simulink model "test"  (R2015b)
settings: Solver=FixedStepDiscrete  StartTime=0.0  StopTime=10.0  FixedStep=0.0005  RelTol=1e-3
undefined symbols (not defined in the file): I_AN03_5V, I_AN11_5V, I_SW11_H, O_SW12_HS1A
libraries: ec5744lib x12, simulink x1
settings Model: Creator=28061  LastModifiedBy=VICTOR7
settings OptimizationCC: DefaultParameterBehavior=Inlined  InlineInvariantSignals=on  ExpressionFolding=off  RollThreshold=9  StateBitsets=on  DataBitsets=on  ZeroExternalMemoryAtStartup=off  ZeroInternalMemoryAtStartup=off  EfficientFloat2IntCast=on  LifeSpan=1
settings DebuggingCC: InheritedTsInSrcMsg=none
settings HardwareCC: ProdBitPerPointer=32  ProdLargestAtomicInteger=Long  ProdLargestAtomicFloat=Double  ProdEndianess=BigEndian  ProdWordSize=32  ProdHWDeviceType=Freescale MPC5500
settings RTWCC: SystemTargetFile=ec5744.tlc  MakeCommand=make_rtw optimized_fixed_point=1  GenerateMakefile=off  TemplateMakefile=ec5744_lcc.tmf  PostCodeGenCommand=ec5744_pst_s2(buildInfo)  Description=Target for EC5744  GenerateReport=on  IncludeHyperlinkInReport=on  LaunchReport=on
settings CodeAppCC: IgnoreCustomStorageClasses=off
settings STFCustomTargetCC: ModelReferenceCompliant=off  ConcurrentExecutionCompliant=off  IncludeMdlTerminateFcn=off  GeneratePreprocessorConditionals=Use local settings  CombineOutputUpdateFcns=on  SuppressErrorStatus=on  ERTCustomFileBanners=on  SupportContinuousTime=off  SupportNonInlinedSFcns=off  SupportVariableSizeSignals=on  MATLABClassNameForMDSCustomization=Simulink.SoftwareTarget.ERTCustomization  CPPClassGenCompliant=off  GRTInterface=off  SystemTargetFile=ec5744.tlc
settings ERTTargetCC: ModelReferenceCompliant=off  ParMdlRefBuildCompliant=off  CompOptLevelCompliant=off  ConcurrentExecutionCompliant=off  IncludeMdlTerminateFcn=off  SuppressErrorStatus=on  ERTFirstTimeCompliant=off  SupportVariableSizeSignals=on  ModelStepFunctionPrototypeControlCompliant=off  CPPClassGenCompliant=off  UseToolchainInfoCompliant=off  GenerateASAP2=on  InlinedParameterPlacement=NonHierarchical  ERTSrcFileBannerTemplate=ec5744_code_template.cgt  ERTHdrFileBannerTemplate=ec5744_code_template.cgt  ERTDataSrcFileTemplate=ec5744_code_template.cgt  ERTDataHdrFileTemplate=ec5744_code_template.cgt  ERTCustomFileTemplate=ec5744_file_process.tlc

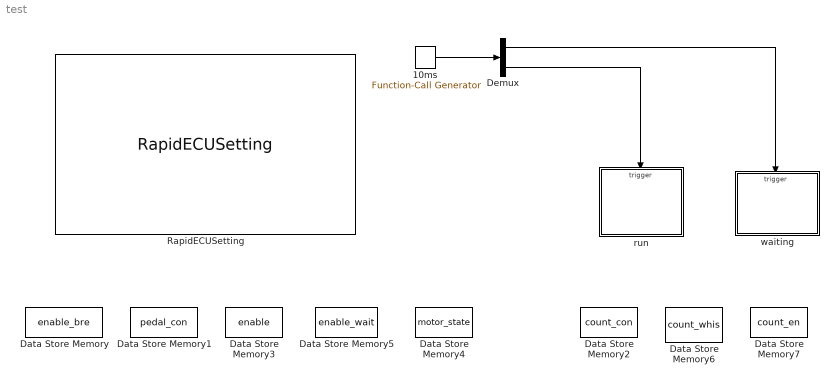
== system test ==
  10ms : simulink/Ports & Subsystems/Function-Call Generator  sample_time=0.01  numberOfIterations=1
  Data Store Memory : DataStoreMemory  DataStoreName=enable_bre  ReadBeforeWriteMsg=warning  WriteAfterWriteMsg=warning  WriteAfterReadMsg=warning
  Data Store Memory1 : DataStoreMemory  DataStoreName=pedal_con  ReadBeforeWriteMsg=warning  WriteAfterWriteMsg=warning  WriteAfterReadMsg=warning
  Data Store Memory2 : DataStoreMemory  DataStoreName=count_con  ReadBeforeWriteMsg=warning  WriteAfterWriteMsg=warning  WriteAfterReadMsg=warning  OutDataTypeStr=double
  Data Store Memory3 : DataStoreMemory  DataStoreName=enable  ReadBeforeWriteMsg=warning  WriteAfterWriteMsg=warning  WriteAfterReadMsg=warning  OutDataTypeStr=boolean
  Data Store Memory4 : DataStoreMemory  DataStoreName=motor_state  ReadBeforeWriteMsg=warning  WriteAfterWriteMsg=warning  WriteAfterReadMsg=warning
  Data Store Memory5 : DataStoreMemory  DataStoreName=enable_wait  ReadBeforeWriteMsg=warning  WriteAfterWriteMsg=warning  WriteAfterReadMsg=warning  OutDataTypeStr=boolean
  Data Store Memory6 : DataStoreMemory  DataStoreName=count_whis  ReadBeforeWriteMsg=warning  WriteAfterWriteMsg=warning  WriteAfterReadMsg=warning  OutDataTypeStr=double
  Data Store Memory7 : DataStoreMemory  DataStoreName=count_en  ReadBeforeWriteMsg=warning  WriteAfterWriteMsg=warning  WriteAfterReadMsg=warning  OutDataTypeStr=double
  Demux : Demux  Outputs=2
  RapidECUSetting : ec5744lib/RapidECU_U3/RapidECUSetting
  run : Subsystem
  waiting : Subsystem
  wires:
  10ms/1 -> Demux/1
  Demux/2 -> run/Trigger
  Demux/1 -> waiting/Trigger

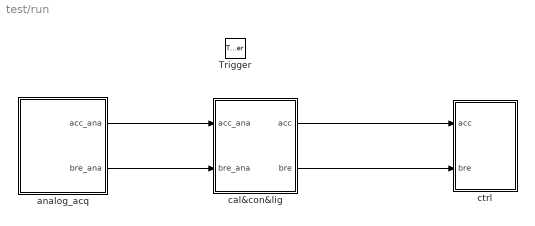
== system test/run ==
  Trigger : TriggerPort  TriggerType=function-call  PortDimensions=1
  analog_acq : Subsystem
  cal&con&lig : Subsystem
  ctrl : Subsystem
  wires:
  analog_acq/2(bre_ana) -> cal&con&lig/2(bre_ana)
  analog_acq/1(acc_ana) -> cal&con&lig/1(acc_ana)
  cal&con&lig/1(acc) -> ctrl/1(acc)
  cal&con&lig/2(bre) -> ctrl/2(bre)

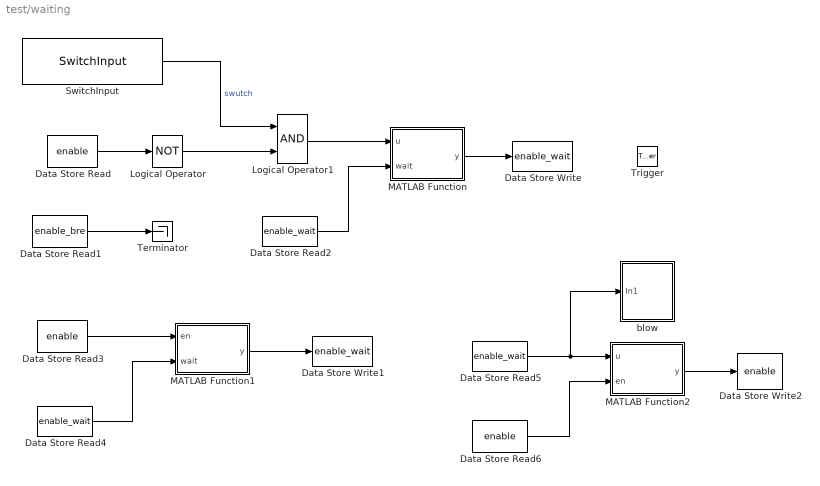
== system test/waiting ==
  Trigger : TriggerPort  TriggerType=function-call  PortDimensions=1
  Data Store Read : DataStoreRead  DataStoreName=enable
  Data Store Read1 : DataStoreRead  DataStoreName=enable_bre
  Data Store Read2 : DataStoreRead  DataStoreName=enable_wait
  Data Store Read3 : DataStoreRead  DataStoreName=enable
  Data Store Read4 : DataStoreRead  DataStoreName=enable_wait
  Data Store Read5 : DataStoreRead  DataStoreName=enable_wait
  Data Store Read6 : DataStoreRead  DataStoreName=enable
  Data Store Write : DataStoreWrite  DataStoreName=enable_wait
  Data Store Write1 : DataStoreWrite  DataStoreName=enable_wait
  Data Store Write2 : DataStoreWrite  DataStoreName=enable
  Logical Operator : Logic  Operator=NOT  AllPortsSameDT=off  OutDataTypeStr=boolean
  Logical Operator1 : Logic  AllPortsSameDT=off  OutDataTypeStr=boolean
  MATLAB Function : MATLAB Function  TreatAsAtomicUnit=on
  MATLAB Function1 : MATLAB Function  TreatAsAtomicUnit=on
  MATLAB Function2 : MATLAB Function  TreatAsAtomicUnit=on
  SwitchInput : ec5744lib/RapidECU_U3/01BasicInput/SwitchInput  channel=44:I_SW11_H  sampletime=-1
  Terminator : Terminator
  blow : Subsystem
  wires:
  Logical Operator/1 -> Logical Operator1/2
  MATLAB Function/1(y) -> Data Store Write/1
  Data Store Read6/1 -> MATLAB Function2/2(en)
  Logical Operator1/1 -> MATLAB Function/1(u)
  Data Store Read2/1 -> MATLAB Function/2(wait)
  Data Store Read3/1 -> MATLAB Function1/1(en)
  Data Store Read5/1 -> blow/1(In1), MATLAB Function2/1(u)
  SwitchInput/1 -> Logical Operator1/1  "swutch"
  Data Store Read4/1 -> MATLAB Function1/2(wait)
  Data Store Read/1 -> Logical Operator/1
  MATLAB Function1/1(y) -> Data Store Write1/1
  MATLAB Function2/1(y) -> Data Store Write2/1
  Data Store Read1/1 -> Terminator/1

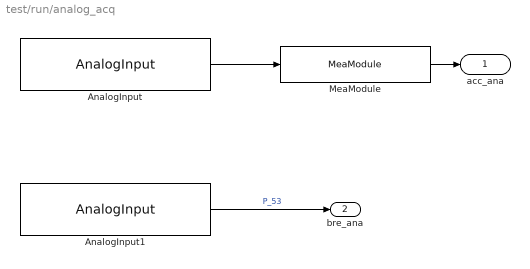
== system test/run/analog_acq ==
  AnalogInput : ec5744lib/RapidECU_U3B/01BasicInput/AnalogInput  channel=52:I_AN03_5V  sampletime=-1
  AnalogInput1 : ec5744lib/RapidECU_U3/01BasicInput/AnalogInput  channel=71:I_AN11_5V  sampletime=-1
  MeaModule : ec5744lib/RapidECU_U3B/07Calibration/MeaModule  signal=ECMeaVar1
  acc_ana : Outport
  bre_ana : Outport  Port=2
  wires:
  AnalogInput1/1 -> bre_ana/1  "P_53"
  MeaModule/1 -> acc_ana/1
  AnalogInput/1 -> MeaModule/1

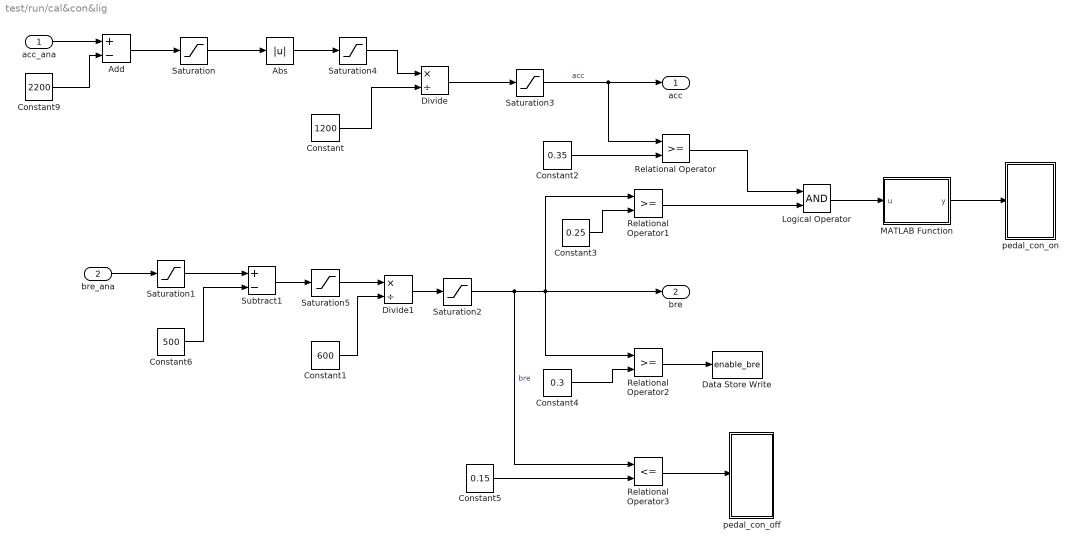
== system test/run/cal&con&lig ==
  acc_ana : Inport
  bre_ana : Inport  Port=2
  Abs : Abs
  Add : Sum  Inputs=+-
  Constant : Constant  Value=1200
  Constant1 : Constant  Value=600
  Constant2 : Constant  Value=0.35
  Constant3 : Constant  Value=0.25
  Constant4 : Constant  Value=0.3
  Constant5 : Constant  Value=0.15
  Constant6 : Constant  Value=500
  Constant9 : Constant  Value=2200
  Data Store Write : DataStoreWrite  DataStoreName=enable_bre
  Divide : Product  Inputs=*/
  Divide1 : Product  Inputs=*/
  Logical Operator : Logic  AllPortsSameDT=off  OutDataTypeStr=boolean
  MATLAB Function : MATLAB Function  TreatAsAtomicUnit=on
  Relational Operator : RelationalOperator  OutDataTypeStr=boolean
  Relational Operator1 : RelationalOperator  OutDataTypeStr=boolean
  Relational Operator2 : RelationalOperator  OutDataTypeStr=boolean
  Relational Operator3 : RelationalOperator  Operator=<=  OutDataTypeStr=boolean
  Saturation : Saturate  UpperLimit=0  LowerLimit=-1200
  Saturation1 : Saturate  UpperLimit=2466  LowerLimit=1533
  Saturation2 : Saturate  UpperLimit=1  LowerLimit=0
  Saturation3 : Saturate  UpperLimit=1  LowerLimit=0
  Saturation4 : Saturate  UpperLimit=1200  LowerLimit=0
  Saturation5 : Saturate  UpperLimit=933  LowerLimit=0
  Subtract1 : Sum  Inputs=+-
  pedal_con_off : Subsystem
  pedal_con_on : Subsystem
  acc : Outport
  bre : Outport  Port=2
  wires:
  Constant3/1 -> Relational Operator1/2
  Relational Operator1/1 -> Logical Operator/2
  Relational Operator/1 -> Logical Operator/1
  Constant5/1 -> Relational Operator3/2
  Relational Operator2/1 -> Data Store Write/1
  Constant4/1 -> Relational Operator2/2
  Relational Operator3/1 -> pedal_con_off/Enable
  MATLAB Function/1(y) -> pedal_con_on/Enable
  Logical Operator/1 -> MATLAB Function/1(u)
  Constant1/1 -> Divide1/2
  Constant/1 -> Divide/2
  Divide1/1 -> Saturation2/1
  Saturation2/1 -> Relational Operator3/1, bre/1, Relational Operator2/1, Relational Operator1/1  "bre"
  Constant2/1 -> Relational Operator/2
  bre_ana/1 -> Saturation1/1
  Divide/1 -> Saturation3/1
  Saturation1/1 -> Subtract1/1
  Constant6/1 -> Subtract1/2
  Subtract1/1 -> Saturation5/1
  Saturation5/1 -> Divide1/1
  Constant9/1 -> Add/2
  acc_ana/1 -> Add/1
  Add/1 -> Saturation/1
  Saturation/1 -> Abs/1
  Abs/1 -> Saturation4/1
  Saturation4/1 -> Divide/1
  Saturation3/1 -> Relational Operator/1, acc/1  "acc"

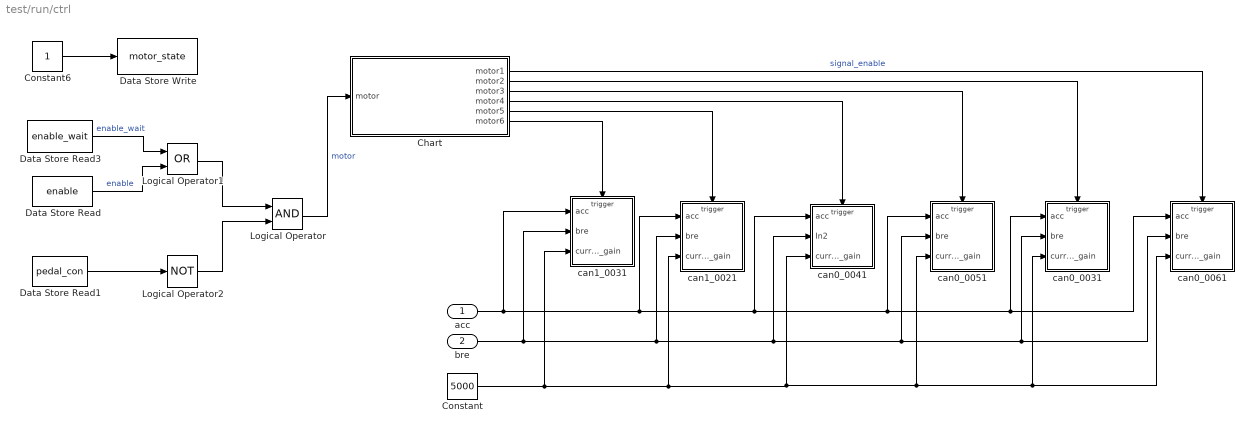
== system test/run/ctrl ==
  acc : Inport
  bre : Inport  Port=2
  Chart : Stateflow chart  TreatAsAtomicUnit=on
  Constant : Constant  Value=5000
  Constant6 : Constant
  Data Store Read : DataStoreRead  DataStoreName=enable
  Data Store Read1 : DataStoreRead  DataStoreName=pedal_con
  Data Store Read3 : DataStoreRead  DataStoreName=enable_wait
  Data Store Write : DataStoreWrite  DataStoreName=motor_state
  Logical Operator : Logic  AllPortsSameDT=off  OutDataTypeStr=boolean
  Logical Operator1 : Logic  Operator=OR  AllPortsSameDT=off  OutDataTypeStr=boolean
  Logical Operator2 : Logic  Operator=NOT  AllPortsSameDT=off  OutDataTypeStr=boolean
  can0_0031 : Subsystem
  can0_0041 : Subsystem
  can0_0051 : Subsystem
  can0_0061 : Subsystem
  can1_0021 : Subsystem
  can1_0031 : Subsystem
  wires:
  Data Store Read3/1 -> Logical Operator1/1  "enable_wait"
  Data Store Read/1 -> Logical Operator1/2  "enable"
  Logical Operator1/1 -> Logical Operator/1
  Data Store Read1/1 -> Logical Operator2/1
  Logical Operator2/1 -> Logical Operator/2
  Constant6/1 -> Data Store Write/1
  acc/1 -> can1_0031/1(acc), can0_0031/1(acc), can0_0061/1(acc), can0_0051/1(acc), can0_0041/1(acc), can1_0021/1(acc)
  bre/1 -> can1_0031/2(bre), can0_0061/2(bre), can0_0031/2(bre), can0_0051/2(bre), can0_0041/2(In2), can1_0021/2(bre)
  Chart/1(motor1) -> can0_0061/Trigger  "signal_enable"
  Chart/2(motor2) -> can0_0031/Trigger
  Chart/3(motor3) -> can0_0051/Trigger
  Chart/4(motor4) -> can0_0041/Trigger
  Logical Operator/1 -> Chart/1(motor)  "motor"
  Constant/1 -> can1_0031/3(current_gain), can0_0061/3(current_gain), can0_0031/3(current_gain), can0_0051/3(current_gain), can0_0041/3("current_gain "), can1_0021/3(current_gain)
  Chart/5(motor5) -> can1_0021/Trigger
  Chart/6(motor6) -> can1_0031/Trigger

== system test/waiting/blow ==
  In1 : Inport
  Chart : Stateflow chart  TreatAsAtomicUnit=on
  Data Type Conversion : DataTypeConversion  OutDataTypeStr=boolean
  PowerDriverSwitch(HS)2 : ec5744lib/RapidECU_U3/02PowerDriverSwitch/PowerDriverSwitch(HS)  channel=114:O_SW12_HS1A  sampletime=-1
  wires:
  In1/1 -> Data Type Conversion/1
  Data Type Conversion/1 -> Chart/1(blow_signal)
  Chart/1(blow_enable) -> PowerDriverSwitch(HS)2/1  "blow"

== system test/run/cal&con&lig/pedal_con_off ==
  Enable : EnablePort
  Constant6 : Constant  Value=0
  Data Store Write1 : DataStoreWrite  DataStoreName=pedal_con
  wires:
  Constant6/1 -> Data Store Write1/1

== system test/run/cal&con&lig/pedal_con_on ==
  Enable : EnablePort
  Constant4 : Constant
  Data Store Write : DataStoreWrite  DataStoreName=pedal_con
  wires:
  Constant4/1 -> Data Store Write/1

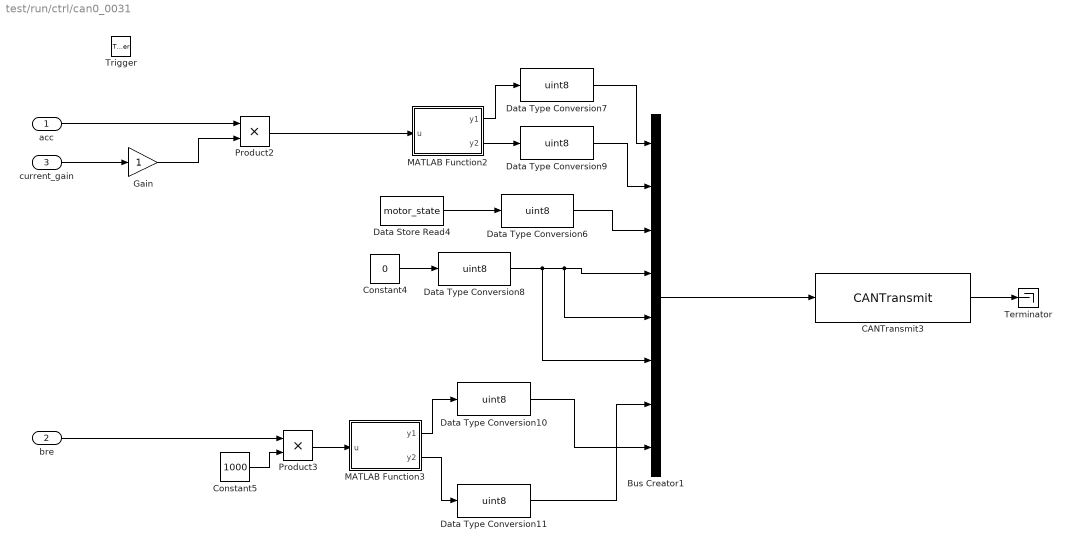
== system test/run/ctrl/can0_0031 ==
  acc : Inport
  bre : Inport  Port=2
  current_gain : Inport  Port=3
  Trigger : TriggerPort  PortDimensions=1
  Bus Creator1 : BusCreator  Inputs=8
  CANTransmit3 : ec5744lib/RapidECU_U3B/04CANCommunication/CANTransmit  canmodule=0  canbuffer=63  canmessageid=hex2dec('0031')  canmessagetype=Standard(11-bit ID)  datalength=8  sampletime=-1
  Constant4 : Constant  Value=0
  Constant5 : Constant  Value=1000
  Data Store Read4 : DataStoreRead  DataStoreName=motor_state
  Data Type Conversion{6..11} (6 alike) : DataTypeConversion  OutDataTypeStr=uint8
  Gain : Gain
  MATLAB Function2 : MATLAB Function  TreatAsAtomicUnit=on
  MATLAB Function3 : MATLAB Function  TreatAsAtomicUnit=on
  Product2 : Product
  Product3 : Product
  Terminator : Terminator
  wires:
  acc/1 -> Product2/1
  MATLAB Function3/2(y2) -> Data Type Conversion11/1
  Constant4/1 -> Data Type Conversion8/1
  Constant5/1 -> Product3/2
  Data Type Conversion8/1 -> Bus Creator1/4, Bus Creator1/5, Bus Creator1/6
  Data Type Conversion6/1 -> Bus Creator1/3
  Data Type Conversion7/1 -> Bus Creator1/1
  Data Store Read4/1 -> Data Type Conversion6/1
  Data Type Conversion9/1 -> Bus Creator1/2
  MATLAB Function2/1(y1) -> Data Type Conversion7/1
  Data Type Conversion11/1 -> Bus Creator1/7
  bre/1 -> Product3/1
  MATLAB Function2/2(y2) -> Data Type Conversion9/1
  Product3/1 -> MATLAB Function3/1(u)
  Data Type Conversion10/1 -> Bus Creator1/8
  Product2/1 -> MATLAB Function2/1(u)
  MATLAB Function3/1(y1) -> Data Type Conversion10/1
  Bus Creator1/1 -> CANTransmit3/1
  current_gain/1 -> Gain/1
  Gain/1 -> Product2/2
  CANTransmit3/1 -> Terminator/1

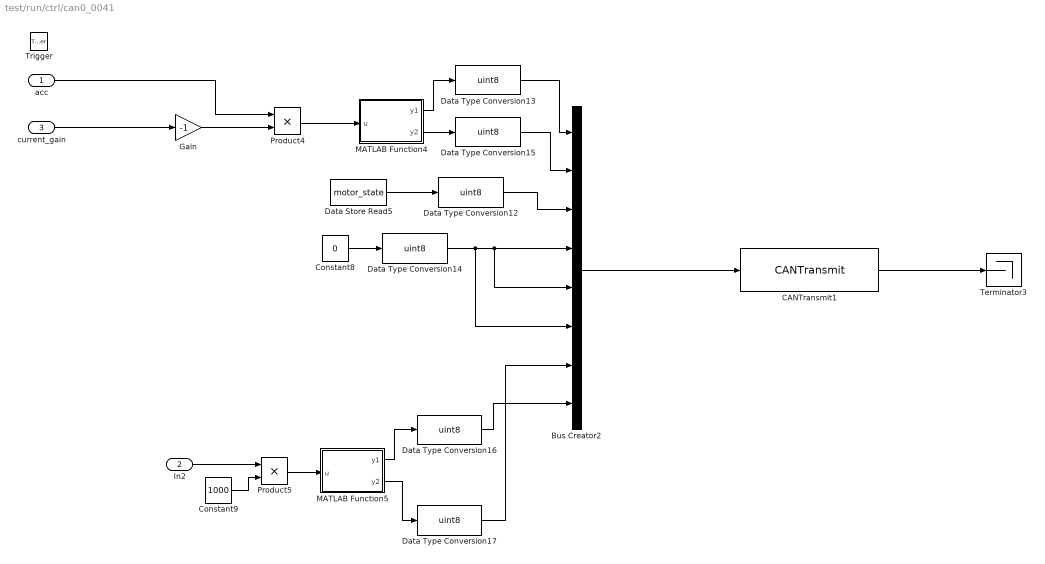
== system test/run/ctrl/can0_0041 ==
  acc : Inport
  In2 : Inport  Port=2
  "current_gain " : Inport  Port=3
  Trigger : TriggerPort  PortDimensions=1
  Bus Creator2 : BusCreator  Inputs=8
  CANTransmit1 : ec5744lib/RapidECU_U3B/04CANCommunication/CANTransmit  canmodule=0  canbuffer=11  canmessageid=hex2dec('0041')  canmessagetype=Standard(11-bit ID)  datalength=8  sampletime=-1
  Constant8 : Constant  Value=0
  Constant9 : Constant  Value=1000
  Data Store Read5 : DataStoreRead  DataStoreName=motor_state
  Data Type Conversion{12..17} (6 alike) : DataTypeConversion  OutDataTypeStr=uint8
  Gain : Gain  Gain=-1
  MATLAB Function4 : MATLAB Function  TreatAsAtomicUnit=on
  MATLAB Function5 : MATLAB Function  TreatAsAtomicUnit=on
  Product4 : Product
  Product5 : Product
  Terminator3 : Terminator
  wires:
  Gain/1 -> Product4/2
  Data Type Conversion12/1 -> Bus Creator2/3
  Constant9/1 -> Product5/2
  Data Type Conversion13/1 -> Bus Creator2/1
  Product4/1 -> MATLAB Function4/1(u)
  MATLAB Function4/1(y1) -> Data Type Conversion13/1
  Constant8/1 -> Data Type Conversion14/1
  Product5/1 -> MATLAB Function5/1(u)
  MATLAB Function4/2(y2) -> Data Type Conversion15/1
  MATLAB Function5/1(y1) -> Data Type Conversion16/1
  MATLAB Function5/2(y2) -> Data Type Conversion17/1
  Data Type Conversion16/1 -> Bus Creator2/8
  Data Type Conversion17/1 -> Bus Creator2/7
  Data Type Conversion15/1 -> Bus Creator2/2
  Data Type Conversion14/1 -> Bus Creator2/4, Bus Creator2/5, Bus Creator2/6
  Data Store Read5/1 -> Data Type Conversion12/1
  CANTransmit1/1 -> Terminator3/1
  Bus Creator2/1 -> CANTransmit1/1
  acc/1 -> Product4/1
  In2/1 -> Product5/1
  "current_gain "/1 -> Gain/1

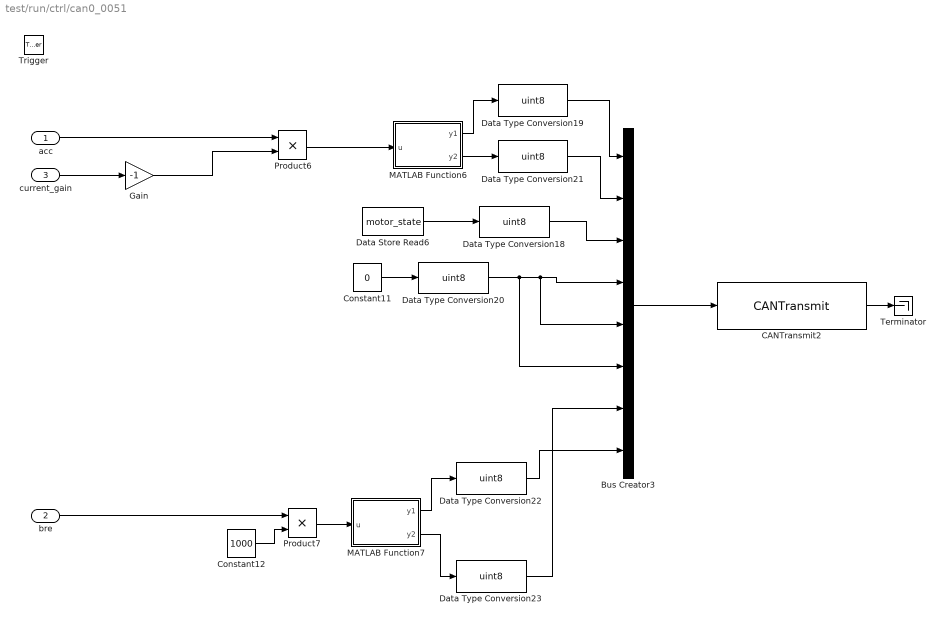
== system test/run/ctrl/can0_0051 ==
  acc : Inport
  bre : Inport  Port=2
  current_gain : Inport  Port=3
  Trigger : TriggerPort  PortDimensions=1
  Bus Creator3 : BusCreator  Inputs=8
  CANTransmit2 : ec5744lib/RapidECU_U3B/04CANCommunication/CANTransmit  canmodule=0  canbuffer=9  canmessageid=hex2dec('0051')  canmessagetype=Standard(11-bit ID)  datalength=8  sampletime=-1
  Constant11 : Constant  Value=0
  Constant12 : Constant  Value=1000
  Data Store Read6 : DataStoreRead  DataStoreName=motor_state
  Data Type Conversion{18..23} (6 alike) : DataTypeConversion  OutDataTypeStr=uint8
  Gain : Gain  Gain=-1
  MATLAB Function6 : MATLAB Function  TreatAsAtomicUnit=on
  MATLAB Function7 : MATLAB Function  TreatAsAtomicUnit=on
  Product6 : Product
  Product7 : Product
  Terminator : Terminator
  wires:
  Data Type Conversion18/1 -> Bus Creator3/3
  Data Type Conversion20/1 -> Bus Creator3/4, Bus Creator3/5, Bus Creator3/6
  Constant12/1 -> Product7/2
  MATLAB Function7/2(y2) -> Data Type Conversion23/1
  Data Type Conversion22/1 -> Bus Creator3/8
  MATLAB Function6/2(y2) -> Data Type Conversion21/1
  Data Type Conversion21/1 -> Bus Creator3/2
  Product7/1 -> MATLAB Function7/1(u)
  MATLAB Function6/1(y1) -> Data Type Conversion19/1
  Data Type Conversion23/1 -> Bus Creator3/7
  Data Type Conversion19/1 -> Bus Creator3/1
  Data Store Read6/1 -> Data Type Conversion18/1
  Constant11/1 -> Data Type Conversion20/1
  MATLAB Function7/1(y1) -> Data Type Conversion22/1
  bre/1 -> Product7/1
  Product6/1 -> MATLAB Function6/1(u)
  acc/1 -> Product6/1
  Bus Creator3/1 -> CANTransmit2/1
  current_gain/1 -> Gain/1
  Gain/1 -> Product6/2
  CANTransmit2/1 -> Terminator/1

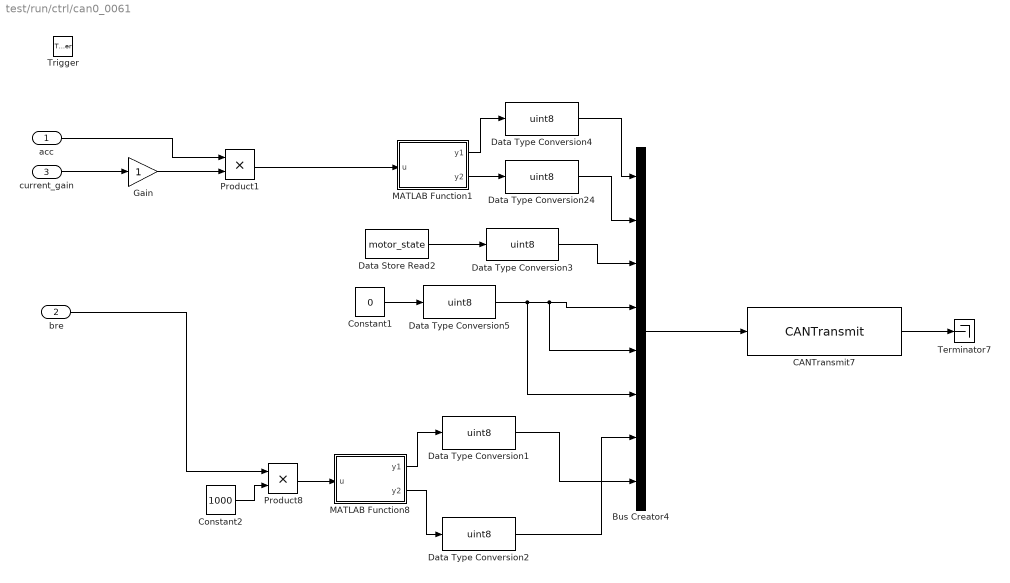
== system test/run/ctrl/can0_0061 ==
  acc : Inport
  bre : Inport  Port=2
  current_gain : Inport  Port=3
  Trigger : TriggerPort  PortDimensions=1
  Bus Creator4 : BusCreator  Inputs=8
  CANTransmit7 : ec5744lib/RapidECU_U3B/04CANCommunication/CANTransmit  canmodule=0  canbuffer=8  canmessageid=hex2dec('0061')  canmessagetype=Standard(11-bit ID)  datalength=8  sampletime=-1
  Constant1 : Constant  Value=0
  Constant2 : Constant  Value=1000
  Data Store Read2 : DataStoreRead  DataStoreName=motor_state
  Data Type Conversion{1..5,24} (6 alike) : DataTypeConversion  OutDataTypeStr=uint8
  Gain : Gain
  MATLAB Function1 : MATLAB Function  TreatAsAtomicUnit=on
  MATLAB Function8 : MATLAB Function  TreatAsAtomicUnit=on
  Product1 : Product
  Product8 : Product
  Terminator7 : Terminator
  wires:
  MATLAB Function8/1(y1) -> Data Type Conversion1/1
  Product1/1 -> MATLAB Function1/1(u)
  Data Type Conversion3/1 -> Bus Creator4/3
  bre/1 -> Product8/1
  MATLAB Function8/2(y2) -> Data Type Conversion2/1
  MATLAB Function1/2(y2) -> Data Type Conversion24/1
  Product8/1 -> MATLAB Function8/1(u)
  Data Type Conversion5/1 -> Bus Creator4/4, Bus Creator4/5, Bus Creator4/6
  Data Type Conversion4/1 -> Bus Creator4/1
  Constant2/1 -> Product8/2
  acc/1 -> Product1/1
  Data Store Read2/1 -> Data Type Conversion3/1
  Constant1/1 -> Data Type Conversion5/1
  Data Type Conversion1/1 -> Bus Creator4/8
  CANTransmit7/1 -> Terminator7/1
  Bus Creator4/1 -> CANTransmit7/1
  MATLAB Function1/1(y1) -> Data Type Conversion4/1
  Data Type Conversion2/1 -> Bus Creator4/7
  Data Type Conversion24/1 -> Bus Creator4/2
  current_gain/1 -> Gain/1
  Gain/1 -> Product1/2

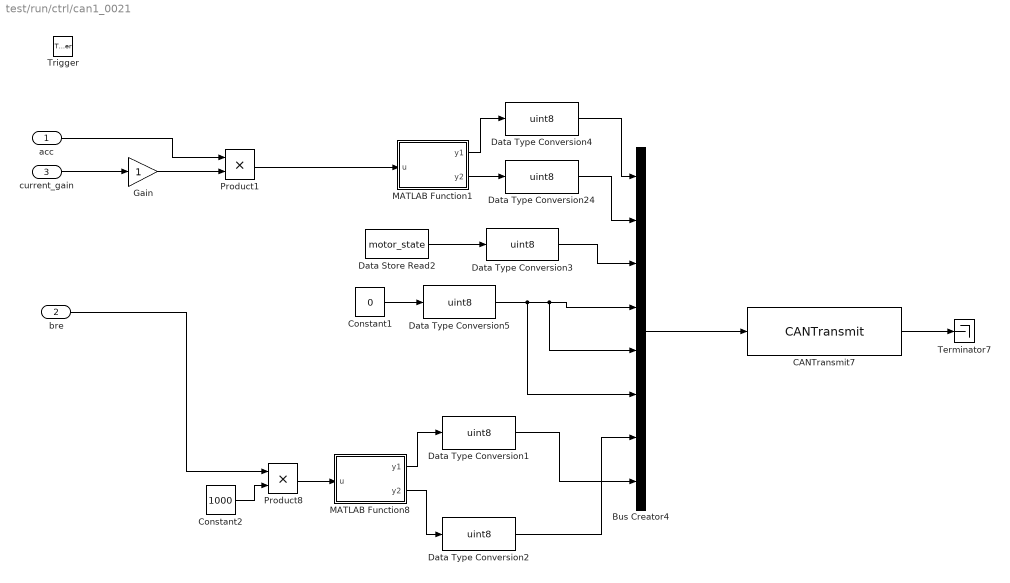
== system test/run/ctrl/can1_0021 ==
  acc : Inport
  bre : Inport  Port=2
  current_gain : Inport  Port=3
  Trigger : TriggerPort  PortDimensions=1
  Bus Creator4 : BusCreator  Inputs=8
  CANTransmit7 : ec5744lib/RapidECU_U3B/04CANCommunication/CANTransmit  canmodule=1  canbuffer=8  canmessageid=hex2dec('0021')  canmessagetype=Standard(11-bit ID)  datalength=8  sampletime=-1
  Constant1 : Constant  Value=0
  Constant2 : Constant  Value=1000
  Data Store Read2 : DataStoreRead  DataStoreName=motor_state
  Data Type Conversion{1..5,24} (6 alike) : DataTypeConversion  OutDataTypeStr=uint8
  Gain : Gain
  MATLAB Function1 : MATLAB Function  TreatAsAtomicUnit=on
  MATLAB Function8 : MATLAB Function  TreatAsAtomicUnit=on
  Product1 : Product
  Product8 : Product
  Terminator7 : Terminator
  wires:
  Gain/1 -> Product1/2
  current_gain/1 -> Gain/1
  Data Type Conversion24/1 -> Bus Creator4/2
  Data Type Conversion2/1 -> Bus Creator4/7
  MATLAB Function1/1(y1) -> Data Type Conversion4/1
  Bus Creator4/1 -> CANTransmit7/1
  CANTransmit7/1 -> Terminator7/1
  Data Type Conversion1/1 -> Bus Creator4/8
  Constant1/1 -> Data Type Conversion5/1
  Data Store Read2/1 -> Data Type Conversion3/1
  acc/1 -> Product1/1
  Constant2/1 -> Product8/2
  Data Type Conversion4/1 -> Bus Creator4/1
  Data Type Conversion5/1 -> Bus Creator4/6, Bus Creator4/5, Bus Creator4/4
  Product8/1 -> MATLAB Function8/1(u)
  MATLAB Function1/2(y2) -> Data Type Conversion24/1
  MATLAB Function8/2(y2) -> Data Type Conversion2/1
  bre/1 -> Product8/1
  Data Type Conversion3/1 -> Bus Creator4/3
  Product1/1 -> MATLAB Function1/1(u)
  MATLAB Function8/1(y1) -> Data Type Conversion1/1

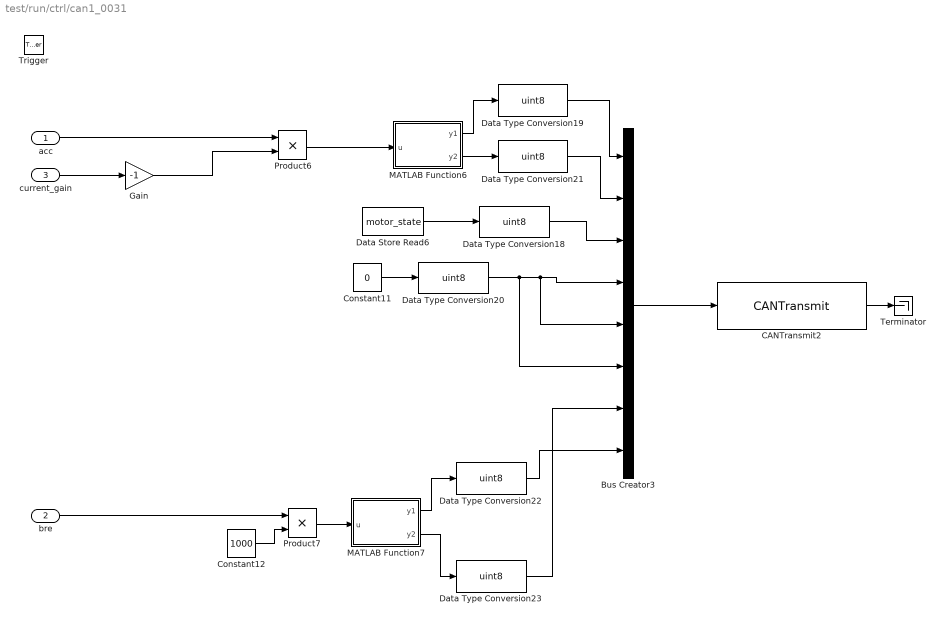
== system test/run/ctrl/can1_0031 ==
  acc : Inport
  bre : Inport  Port=2
  current_gain : Inport  Port=3
  Trigger : TriggerPort  PortDimensions=1
  Bus Creator3 : BusCreator  Inputs=8
  CANTransmit2 : ec5744lib/RapidECU_U3B/04CANCommunication/CANTransmit  canmodule=1  canbuffer=9  canmessageid=hex2dec('0031')  canmessagetype=Standard(11-bit ID)  datalength=8  sampletime=-1
  Constant11 : Constant  Value=0
  Constant12 : Constant  Value=1000
  Data Store Read6 : DataStoreRead  DataStoreName=motor_state
  Data Type Conversion{18..23} (6 alike) : DataTypeConversion  OutDataTypeStr=uint8
  Gain : Gain  Gain=-1
  MATLAB Function6 : MATLAB Function  TreatAsAtomicUnit=on
  MATLAB Function7 : MATLAB Function  TreatAsAtomicUnit=on
  Product6 : Product
  Product7 : Product
  Terminator : Terminator
  wires:
  CANTransmit2/1 -> Terminator/1
  Gain/1 -> Product6/2
  current_gain/1 -> Gain/1
  Bus Creator3/1 -> CANTransmit2/1
  acc/1 -> Product6/1
  Product6/1 -> MATLAB Function6/1(u)
  bre/1 -> Product7/1
  MATLAB Function7/1(y1) -> Data Type Conversion22/1
  Constant11/1 -> Data Type Conversion20/1
  Data Store Read6/1 -> Data Type Conversion18/1
  Data Type Conversion19/1 -> Bus Creator3/1
  Data Type Conversion23/1 -> Bus Creator3/7
  MATLAB Function6/1(y1) -> Data Type Conversion19/1
  Product7/1 -> MATLAB Function7/1(u)
  Data Type Conversion21/1 -> Bus Creator3/2
  MATLAB Function6/2(y2) -> Data Type Conversion21/1
  Data Type Conversion22/1 -> Bus Creator3/8
  MATLAB Function7/2(y2) -> Data Type Conversion23/1
  Constant12/1 -> Product7/2
  Data Type Conversion20/1 -> Bus Creator3/6, Bus Creator3/5, Bus Creator3/4
  Data Type Conversion18/1 -> Bus Creator3/3

== matlab function test/waiting/MATLAB Function ==
  data: u input; y output; wait input; count_whis data_store_memory
function y = fcn(u,wait)
%#codegen
global count_whis
if u==0
    count_whis=0;
else
    count_whis=count_whis+1;
end

if count_whis>=20
    count_whis=20;
    y=true;
else
    y=wait;
end

== matlab function test/run/cal&con&lig/MATLAB Function ==
  data: u input; y output; count_con data_store_memory
function y = fcn(u)
%#codegen
global count_con
if u==1
    count_con=count_con+1;
else
    count_con=0;
end

if count_con>=50
    y= true ;
    count_con=50;
else
    y= false ;
end

== matlab function test/waiting/MATLAB Function1 ==
  data: en input; y output; wait input
function y = fcn(en,wait)
%#codegen
if en == true
    y = false;
else
    y = wait;
end

== matlab function test/waiting/MATLAB Function2 ==
  data: u input; en input; y output; count_en data_store_memory
function y = fcn(u,en)
%#codegen
global count_en
if u==1
    count_en=count_en+1;
else
    count_en=0;
end

if count_en>=260
    y= true ;
    count_en=260;
else
    y=en;
end

== matlab function test/run/ctrl/can0_0061/MATLAB Function1 ==
  data: u input; y1 output; y2 output
function [y1,y2] = fcn(u)

if u < 256
    y1 = u;
    y2 = 0;
else
    temp = dec2hex(u);
%     temp = reverse(temp);
    v = size(temp);
    if v(2) > 3
        y1 = [temp(3),temp(4)];
        y1 = hex2dec(y1);
        y2 = [temp(1),temp(2)];
        y2 = hex2dec(y2);
    else
        y1 = [temp(2),temp(3)];
        y1 = hex2dec(y1);
        y2 = temp(1);
        y2 = hex2dec(y2);
    end
end

== matlab function test/run/ctrl/can0_0061/MATLAB Function8 ==
  data: u input; y1 output; y2 output
function [y1,y2] = fcn(u)

if u < 256
    y1 = u;
    y2 = 0;
else
    temp = dec2hex(u);
%     temp = reverse(temp);
    v = size(temp);
    if v(2) > 3
        y1 = [temp(3),temp(4)];
        y1 = hex2dec(y1);
        y2 = [temp(1),temp(2)];
        y2 = hex2dec(y2);
    else
        y1 = [temp(2),temp(3)];
        y1 = hex2dec(y1);
        y2 = temp(1);
        y2 = hex2dec(y2);
    end
end

== matlab function test/run/ctrl/can0_0031/MATLAB Function2 ==
  data: u input; y1 output; y2 output
function [y1,y2] = fcn(u)

if u < 256
    y1 = u;
    y2 = 0;
else
    temp = dec2hex(u);
%     temp = reverse(temp);
    v = size(temp);
    if v(2) > 3
        y1 = [temp(3),temp(4)];
        y1 = hex2dec(y1);
        y2 = [temp(1),temp(2)];
        y2 = hex2dec(y2);
    else
        y1 = [temp(2),temp(3)];
        y1 = hex2dec(y1);
        y2 = temp(1);
        y2 = hex2dec(y2);
    end
end

== matlab function test/run/ctrl/can0_0031/MATLAB Function3 ==
  data: u input; y1 output; y2 output
function [y1,y2] = fcn(u)

if u < 256
    y1 = u;
    y2 = 0;
else
    temp = dec2hex(u);
%     temp = reverse(temp);
    v = size(temp);
    if v(2) > 3
        y1 = [temp(3),temp(4)];
        y1 = hex2dec(y1);
        y2 = [temp(1),temp(2)];
        y2 = hex2dec(y2);
    else
        y1 = [temp(2),temp(3)];
        y1 = hex2dec(y1);
        y2 = temp(1);
        y2 = hex2dec(y2);
    end
end

== matlab function test/run/ctrl/can0_0041/MATLAB Function4 ==
  data: u input; y1 output; y2 output
function [y1,y2] = fcn(u)
if u==0
    u=0;
else
    temp = dec2bin(u+2^16,16);
    u = bin2dec(temp);
end

if u < 256
    y1 = u;
    y2 = 0;
else
    temp = dec2hex(u);
%     temp = reverse(temp);
    v = size(temp);
    if v(2) > 3
        y1 = [temp(3),temp(4)];
        y1 = hex2dec(y1);
        y2 = [temp(1),temp(2)];
        y2 = hex2dec(y2);
    else
        y1 = [temp(2),temp(3)];
        y1 = hex2dec(y1);
        y2 = temp(1);
        y2 = hex2dec(y2);
    end
end

== matlab function test/run/ctrl/can0_0041/MATLAB Function5 ==
  data: u input; y1 output; y2 output
function [y1,y2] = fcn(u)

if u < 256
    y1 = u;
    y2 = 0;
else
    temp = dec2hex(u);
%     temp = reverse(temp);
    v = size(temp);
    if v(2) > 3
        y1 = [temp(3),temp(4)];
        y1 = hex2dec(y1);
        y2 = [temp(1),temp(2)];
        y2 = hex2dec(y2);
    else
        y1 = [temp(2),temp(3)];
        y1 = hex2dec(y1);
        y2 = temp(1);
        y2 = hex2dec(y2);
    end
end

== matlab function test/run/ctrl/can0_0051/MATLAB Function6 ==
  data: u input; y1 output; y2 output
function [y1,y2] = fcn(u)
if u==0
    u=0;
else
    temp = dec2bin(u+2^16,16);
    u = bin2dec(temp);
end

if u < 256
    y1 = u;
    y2 = 0;
else
    temp = dec2hex(u);
%     temp = reverse(temp);
    v = size(temp);
    if v(2) > 3
        y1 = [temp(3),temp(4)];
        y1 = hex2dec(y1);
        y2 = [temp(1),temp(2)];
        y2 = hex2dec(y2);
    else
        y1 = [temp(2),temp(3)];
        y1 = hex2dec(y1);
        y2 = temp(1);
        y2 = hex2dec(y2);
    end
end

== matlab function test/run/ctrl/can0_0051/MATLAB Function7 ==
  data: u input; y1 output; y2 output
function [y1,y2] = fcn(u)

if u < 256
    y1 = u;
    y2 = 0;
else
    temp = dec2hex(u);
%     temp = reverse(temp);
    v = size(temp);
    if v(2) > 3
        y1 = [temp(3),temp(4)];
        y1 = hex2dec(y1);
        y2 = [temp(1),temp(2)];
        y2 = hex2dec(y2);
    else
        y1 = [temp(2),temp(3)];
        y1 = hex2dec(y1);
        y2 = temp(1);
        y2 = hex2dec(y2);
    end
end

== stateflow chart test/run/ctrl/Chart ==
  state en_ready_true
    entry:
    motor1 = false;
    motor2 = false;
    motor3 = false;
    motor4 = false;
    motor5 = false;
    motor6 = false;
  state mentry_1
    entry:
    motor6=false;
    motor1=true;
  state mentry_2
    entry:
    motor1=false;
    motor2=true;
  state mentry_3
    entry:
    motor2=false;
    motor3=true;
  state mentry_6
    entry:
    motor5=false;
    motor6=true;
  state mentry_5
    entry:
    motor4=false;
    motor5=true;
  state mentry_4
    entry:
    motor3=false;
    motor4=true;
  (default) -> en_ready_true
  mentry_2 -> mentry_3 : after(20,msec)
  mentry_1 -> mentry_2 : after(20,msec)
  en_ready_true -> mentry_1 : [motor==true]
  mentry_6 -> mentry_1 : after(20,msec)
  mentry_3 -> mentry_4 : after(20,msec)
  mentry_5 -> mentry_6 : after(20,msec)
  mentry_4 -> mentry_5 : after(20,msec)
  data: motor1 output; motor2 output; motor3 output; motor4 output; motor input; motor5 output; motor6 output

== stateflow chart test/waiting/blow/Chart ==
  state pre
    entry:blow_enable=false;
  state ing
    entry:blow_enable=true;
  state ready
    entry:blow_enable=false;
  (default) -> pre
  pre -> ing : [blow_signal == 1]
  ing -> ready : after(3,sec)
  data: blow_signal input; blow_enable output

== matlab function test/run/ctrl/can1_0031/MATLAB Function6 ==
  data: u input; y1 output; y2 output
function [y1,y2] = fcn(u)
if u==0
    u=0;
else
    temp = dec2bin(u+2^16,16);
    u = bin2dec(temp);
end

if u < 256
    y1 = u;
    y2 = 0;
else
    temp = dec2hex(u);
%     temp = reverse(temp);
    v = size(temp);
    if v(2) > 3
        y1 = [temp(3),temp(4)];
        y1 = hex2dec(y1);
        y2 = [temp(1),temp(2)];
        y2 = hex2dec(y2);
    else
        y1 = [temp(2),temp(3)];
        y1 = hex2dec(y1);
        y2 = temp(1);
        y2 = hex2dec(y2);
    end
end

== matlab function test/run/ctrl/can1_0031/MATLAB Function7 ==
  data: u input; y1 output; y2 output
function [y1,y2] = fcn(u)

if u < 256
    y1 = u;
    y2 = 0;
else
    temp = dec2hex(u);
%     temp = reverse(temp);
    v = size(temp);
    if v(2) > 3
        y1 = [temp(3),temp(4)];
        y1 = hex2dec(y1);
        y2 = [temp(1),temp(2)];
        y2 = hex2dec(y2);
    else
        y1 = [temp(2),temp(3)];
        y1 = hex2dec(y1);
        y2 = temp(1);
        y2 = hex2dec(y2);
    end
end

== matlab function test/run/ctrl/can1_0021/MATLAB Function1 ==
  data: u input; y1 output; y2 output
function [y1,y2] = fcn(u)

if u < 256
    y1 = u;
    y2 = 0;
else
    temp = dec2hex(u);
%     temp = reverse(temp);
    v = size(temp);
    if v(2) > 3
        y1 = [temp(3),temp(4)];
        y1 = hex2dec(y1);
        y2 = [temp(1),temp(2)];
        y2 = hex2dec(y2);
    else
        y1 = [temp(2),temp(3)];
        y1 = hex2dec(y1);
        y2 = temp(1);
        y2 = hex2dec(y2);
    end
end

== matlab function test/run/ctrl/can1_0021/MATLAB Function8 ==
  data: u input; y1 output; y2 output
function [y1,y2] = fcn(u)

if u < 256
    y1 = u;
    y2 = 0;
else
    temp = dec2hex(u);
%     temp = reverse(temp);
    v = size(temp);
    if v(2) > 3
        y1 = [temp(3),temp(4)];
        y1 = hex2dec(y1);
        y2 = [temp(1),temp(2)];
        y2 = hex2dec(y2);
    else
        y1 = [temp(2),temp(3)];
        y1 = hex2dec(y1);
        y2 = temp(1);
        y2 = hex2dec(y2);
    end
end
